simulink model "mj_res_test"  (R2025a)
settings: Solver=VariableStepAuto  StartTime=0.0  StopTime=2  RelTol=1e-3
undefined symbols (not defined in the file or in its folder): gray, zfar, znear
libraries: mjLib x3
settings Model: PacingRate=8  Creator=MuJoCo Simulink Blockset  LastModifiedBy=turbo
settings OptimizationCC: ReuseModelBlockBuffer=off
settings ModelReferenceCC: EnableRefExpFcnMdlSchedulingChecks=on
settings SFSimCC: SimTargetLang=C++  SimDLTargetLibrary=mkl-dnn
settings RTWCC: GPUComputeCapability=3.5

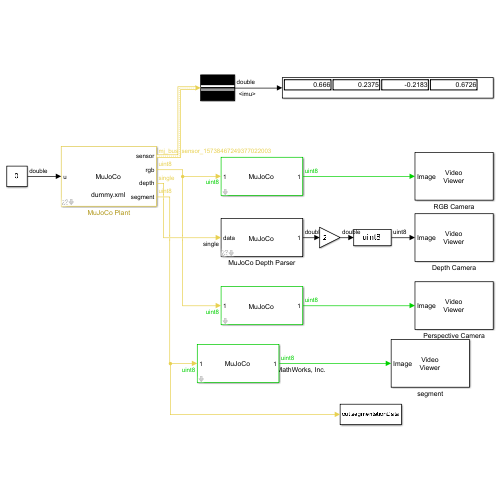
[thumbnail: Simulink's stored preview of the top-level diagram]
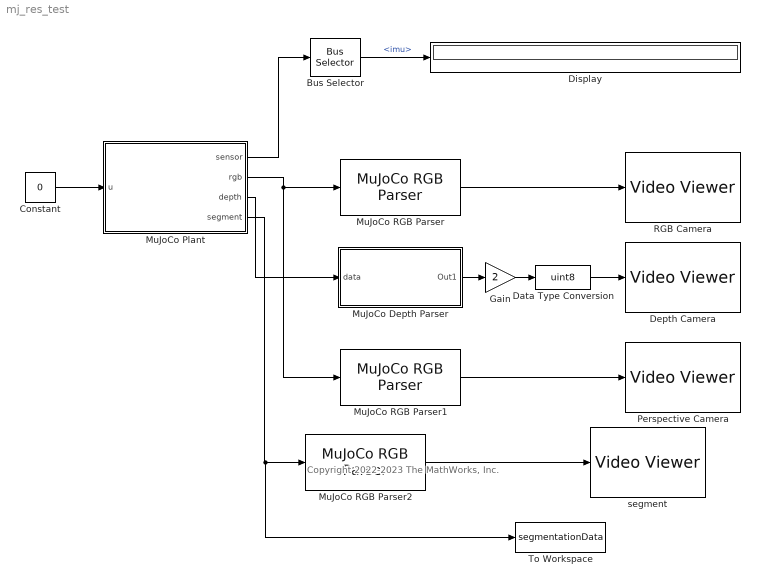
== system mj_res_test ==
  note: Copyright 2022-2023 The MathWorks, Inc.
  Bus Selector : BusSelector  OutputSignals=imu
  Constant : Constant  Value=0
  Data Type Conversion : DataTypeConversion  OutDataTypeStr=uint8  SaturateOnIntegerOverflow=off  RndMeth=Floor
  Depth Camera : VideoViewer  colormapValue=gray(256)  FigPos=[1776 885 418 465]
  Display : Display
  Gain : Gain  Gain=2
  MuJoCo Depth Parser : Subsystem  AncestorBlock=mjLib/MuJoCo Depth Parser  mask{inputBusType=mj_bus_rgb_3624495926710663437, selectedCamera=camera, imageRows=480, imageCols=640, startingIndex=307201, endingIndex=614400, orthographic_enable=on}
      mask prompts: inputBusType "Input Type"; selectedCamera "Select Camera"; orthographic_enable "Orthographic Camera"
      mask TypeOptions inputBusType: mj_bus_rgb_13812558253653659140
      mask Callback inputBusType:
      | inputBusType = get_param(gcb, 'inputBusType');
      | 
      | inputStruct = Simulink.Bus.createMATLABStruct(inputBusType);
      | 
      | mo = Simulink.Mask.get(gcb);
      | mo.Parameters(2).TypeOptions = fieldnames(inputStruct);
      mask TypeOptions selectedCamera: PerspectiveCamera | camera
      mask Callback selectedCamera:
      | inputBusType = get_param(gcb, 'inputBusType');
      | selectedCamera = get_param(gcb, 'selectedCamera');
      | 
      | inputStruct = Simulink.Bus.createMATLABStruct(inputBusType);
      | imageSize = size(inputStruct.(selectedCamera));
      | 
      | imageRows = imageSize(1);
      | imageCols = imageSize(2);
      | 
      | set_param(gcb, 'imageRows', num2str(imageRows));
      | set_param(gcb, 'imageCols', num2str(imageCols));
      | assignin('base', 'imageRows',imageRows);
      | assignin('base', 'imageCols',imageCols);
      | 
      | fields = fieldnames(inputStruct);
      | [~, camIndex] = ismember(selectedCamera, fields);
      | 
      | startingIndex = 1;
      | for i=1:(camIndex-1)
      |     imageSize = size(inputStruct.(fields{i}));
      |     startingIndex = startingIndex + imageSize(1)*imageSize(2);
      | end
      | endingIndex = startingIndex+imageSize(1) * imageSize(2) - 1;
      | 
      | set_param(gcb, 'startingIndex', num2str(startingIndex));
      | set_param(gcb, 'endingIndex', num2str(endingIndex));
      mask DialogControl Control2 Prompt: Refresh
      mask DialogControl Control2 Callback:
      | mo = Simulink.Mask.get(gcb);
      | mo.Parameters(1).TypeOptions = evalin('base', "who('mj_bus_rgb*')");
      mask Display:
      | color('black')
      | text(0.5, 0.5, 'MuJoCo', 'horizontalAlignment', 'center')
  MuJoCo Plant : Subsystem  AncestorBlock=mjLib/MuJoCo Plant  VariantControl=rgbOutOption  mask(MuJoCo Plant){controlBus=[], sensorBus=mj_bus_sensor_7979902499018342666, controlLength=[], sensorLength=[], rgbLength=[], depthLength=[], segLength=[], sampleTime=0.005, xmlFileRel=dummy.xml, xmlFile=dummy.xml, renderingType=Local, vsync=off, visualFPS=60, zoomLevel=1, keyframeName='home', znear=0.059256, zfar=296.2816, cameraSampleTime=0.020, rgbOutOption=on, depthOutOption=on, segmentationOutOption=on, customWidth=640, customHeight=480, specificCameraIndex=-1, controlInterfaceType=Vector}
      mask prompts: renderingType "Type"; visualFPS "FPS"; zoomLevel "Zoom"; keyframeName "Key Frame"; cameraSampleTime "Sample Time"; rgbOutOption "RGB Output"; depthOutOption "Depth Output"; segmentationOutOption "Segmentation Output"; customWidth "Width"; customHeight "Height"; specificCameraIndex "Camera Index"; controlInterfaceType "Interface"
      mask help:
      | This block provides an interface to MuJoCo™ physics engine.
      | It sets control inputs, steps the engine and outputs sensor/camera.
      |
      | Inputs, sensors, cameras and sample time information is obtained from the model XML.
      |
      | Control inputs are provided either as a non-virtual bus or vector.
      | Sensors are output as a non-virtual bus.
      | Camera data is output as a vector which can be decoded using MuJoCo RGB/Depth Parser blocks.
      mask init:
      | [controlBus, sensorBus, rgbBus, depthBus, segmentationBus, dataLengths] = mj_initbus(xmlFile);
      |     controlLength = double(dataLengths(1));
      |     sensorLength = double(dataLengths(2));
      |     rgbLength = double(dataLengths(3));
      |     depthLength = double(dataLengths(4));
      |     segLength = double(dataLengths(5));
      |     mj_maskinit;
      mask Callback xmlFileRel:
      | relpath = get_param(gcb, 'xmlFileRel');
      | 
      | abspath = which(relpath);
      | if isempty(abspath)
      |     abspath = relpath;
      | end
      | set_param(gcb, 'xmlFile', abspath);
      mask TypeOptions renderingType: Local | Global | None
      mask TypeOptions controlInterfaceType: Bus | Vector
      mask DialogControl Container3 Prompt: Model Info
      mask DialogControl controlBusText Prompt: Control Vector Type: [armMotor]
      mask DialogControl sensorBusText Prompt: Sensor Bus Type: mj_bus_sensor_15738467249377022003
      mask DialogControl rgbBusText Prompt: RGB Bus Type: mj_bus_rgb_3624495926710663437
      mask DialogControl depthBusText Prompt: Depth Bus Type: mj_bus_depth_3624495926710663437
      mask DialogControl segmentationBusText Prompt: Segmentation Bus Type: mj_bus_segmentation_3624495926710663437
      mask DialogControl sampleTimeText Prompt: Sample Time: 0.005
      mask DialogControl Container10 Prompt: Model
      mask DialogControl getFileButton Prompt: Browse
      mask DialogControl getFileButton Callback:
      | oldPath = get_param(gcb, 'xmlFile');
      | [file, path] = uigetfile({'*.xml;*.urdf'}, 'File Selector', oldPath);
      | if file~=0
      |     xml = fullfile(path, file);
      |     set_param(gcb, 'xmlFileRel', xml);
      | end
      mask DialogControl testStandaloneButton Prompt: Test
      mask DialogControl testStandaloneButton Callback:
      | % Get the absolute path of the XML file from the block parameter
      |     xmlFile = get_param(gcb, 'xmlFile');
      | 
      |     % Check if the XML file exists
      |     if ~isfile(xmlFile)
      |         error('The specified XML file does not exist: %s', xmlFile);
      |     end
      | 
      |     % Programmatically find the path to simulate.exe
      |     currentFilePath = mfilename('fullpath');
      |     [currentDir, ~, ~] = fileparts(currentFilePath);
      |     mujocoBinPath = fullfile(currentDir, '..', 'lib', 'win64', 'mujoco', 'bin');
      |     simulateExe = fullfile(mujocoBinPath, 'simulate.exe');
      | 
      |     % Check if simulate.exe exists
      |     if ~isfile(simulateExe)
      |         error('simulate.exe not found in the MuJoCo installation folder: %s', simulateExe);
      |     end
      | 
      |     % Run simulate.exe with the XML file as an argument
      |     command = sprintf('"%s" "%s"', simulateExe, xmlFile);
      |     disp(['Running command: ', command]);
      |     status = system(command);
      | 
      |     % Check the status of the command
      |     if status ~= 0
      |         error('Failed to run simulate.exe. Please check the XML file and MuJoCo installation.');
      |     else
      |         disp('Simulation completed successfully.');
      |     end
      mask DialogControl Container12 Prompt: Rendering
      mask DialogControl Control11 Prompt: Rendering thread is common to all MuJoCo blocks and is used for rendering visualizer window along with all cameras
      mask DialogControl Container9 Prompt: Visualizer
      mask DialogControl Control10 Prompt: Visualizer renders frames at specified FPS. Display buffer swap timing is controlled separately via vsync option.
      mask DialogControl renderingType Tooltip: Local rendering creates a unique window for each MuJoCo block. Global tries to merge different block visuals into one window. None disables visualization
      mask DialogControl Container11 Prompt: Options
      mask DialogControl vsync Tooltip: Vsync blocks rendering thread until the monitor is ready to show the next frame. This prevents screen tearing effect. Vsync can slow down everything including physics loop.
      mask DialogControl visualFPS Tooltip: If Vsync is disabled, specify the FPS to show visuals at.
      mask DialogControl Container13 Prompt: Camera
      mask DialogControl Control9 Prompt: Camera rendering runs in lockstep with physics engine.
      mask DialogControl rgbOutOption Tooltip: Render RGB camera
      mask DialogControl depthOutOption Tooltip: Disable depth buffer processing to improve simulation speed.
      mask DialogControl segmentationOutOption Tooltip: Enable segmentation image output using object IDs for each pixel.
      mask DialogControl Container7 Prompt: Control Inputs
      mask Display:
      | color('black')
      | text(0.5, 0.5, 'MuJoCo', 'horizontalAlignment', 'center')
      | [~, nameText, ext] = fileparts(get_param(gcb, 'xmlFile'));
      | text(0.5, 0.2, [nameText, ext], 'horizontalAlignment', 'center')
  MuJoCo RGB Parser : mjLib/MuJoCo RGB Parser  inputBusType=mj_bus_rgb_3624495926710663437  selectedCamera=camera  imageRows=480  imageCols=640  startingIndex=921601  endingIndex=1843200
      settings: SourceProductName=MuJoCo Simulator
  MuJoCo RGB Parser1 : mjLib/MuJoCo RGB Parser  inputBusType=mj_bus_rgb_3624495926710663437  selectedCamera=PerspectiveCamera  imageRows=480  imageCols=640  startingIndex=1  endingIndex=921600
      settings: SourceProductName=MuJoCo Simulator
  MuJoCo RGB Parser2 : mjLib/MuJoCo RGB Parser  inputBusType=mj_bus_rgb_3624495926710663437  selectedCamera=PerspectiveCamera  imageRows=480  imageCols=640  startingIndex=1  endingIndex=921600
      settings: SourceProductName=MuJoCo Simulator
  Perspective Camera : VideoViewer  colormapValue=gray(256)  FigPos=[551 807 418 304]
  RGB Camera : VideoViewer  FigPos=[1323 530 418 332]
  To Workspace : ToWorkspace  VariableName=segmentationData  SaveFormat=Timeseries  SampleTime=-1
  segment : VideoViewer  FigPos=[-428 1519 1118 553]
  wires:
  MuJoCo Plant/2(rgb) -> MuJoCo RGB Parser1/1, MuJoCo RGB Parser/1
  MuJoCo Plant/3(depth) -> MuJoCo Depth Parser/1(data)
  MuJoCo Plant/1(sensor) -> Bus Selector/1
  Bus Selector/1 -> Display/1  "<imu>"
  MuJoCo RGB Parser/1 -> RGB Camera/1
  MuJoCo Depth Parser/1(Out1) -> Gain/1
  Constant/1 -> MuJoCo Plant/1(u)
  Data Type Conversion/1 -> Depth Camera/1
  Gain/1 -> Data Type Conversion/1
  MuJoCo RGB Parser1/1 -> Perspective Camera/1
  MuJoCo RGB Parser2/1 -> segment/1
  MuJoCo Plant/4(segment) -> To Workspace/1, MuJoCo RGB Parser2/1

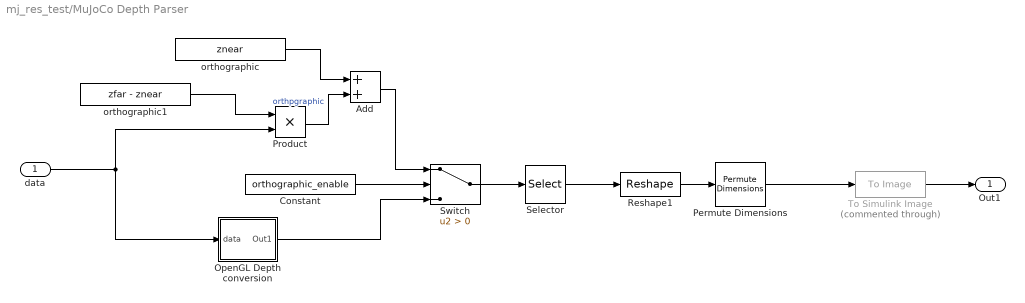
== system mj_res_test/MuJoCo Depth Parser ==
  data : Inport
  Add : Sum
  Constant : Constant  Value=orthographic_enable
  OpenGL Depth conversion : Subsystem
  Permute Dimensions : PermuteDimensions  Order=[3 2 1]
  Product : Product
  Reshape1 : Reshape  OutputDimensionality=Customize  OutputDimensions=[1,imageCols, imageRows]
  Selector : Selector  IndexOptions=Index vector (dialog)  Indices=startingIndex:endingIndex  OutputSizes=1
  Switch : Switch  Criteria=u2 > Threshold  SaturateOnIntegerOverflow=off  InputSameDT=off
  To Simulink Image : ToImage  Commented=through  OutDataTypeStr=Simulink.ImageType(imageRows,imageCols,1,'ColorFormat','Grayscale','Layout','ColumnMajor','ClassUnderlying','single')
  orthographic : Constant  Value=znear
  orthographic1 : Constant  Value=zfar - znear
  Out1 : Outport
  wires:
  Permute Dimensions/1 -> To Simulink Image/1
  To Simulink Image/1 -> Out1/1
  Selector/1 -> Reshape1/1
  data/1 -> OpenGL Depth conversion/1(data), Product/2
  Reshape1/1 -> Permute Dimensions/1
  Switch/1 -> Selector/1
  Constant/1 -> Switch/2
  orthographic1/1 -> Product/1
  OpenGL Depth conversion/1(Out1) -> Switch/3
  orthographic/1 -> Add/1
  Product/1 -> Add/2  "orthpgraphic"
  Add/1 -> Switch/1

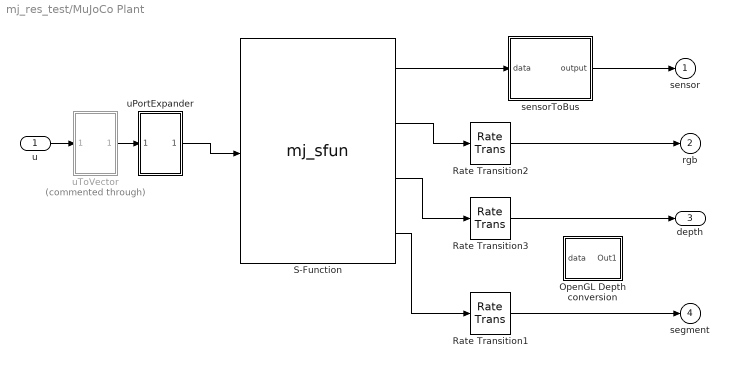
== system mj_res_test/MuJoCo Plant ==
  u : Inport  PortDimensions="[1  1]"
  OpenGL Depth conversion : Subsystem  AncestorBlock=mjLib/MuJoCo Depth Parser/OpenGL Depth conversion
  Rate Transition1 : RateTransition  OutPortSampleTime=cameraSampleTime
  Rate Transition2 : RateTransition  OutPortSampleTime=cameraSampleTime
  Rate Transition3 : RateTransition  OutPortSampleTime=cameraSampleTime
  S-Function : S-Function  FunctionName=mj_sfun  Parameters=xmlFile, renderingType, controlLength, sensorLength, rgbLength, depthLength, vsync, visualFPS, cameraSampleTime, sampleTime, zoomLevel,keyframeName, customWidth, customHeight, specificCameraIndex  SFunctionDeploymentMode=off  EnableBusSupport=off
  sensorToBus : Subsystem
  uPortExpander : Subsystem
  uToVector : Subsystem  Commented=through
  sensor : Outport
  rgb : Outport  Port=2
  depth : Outport  Port=3
  segment : Outport  Port=4
  wires:
  Rate Transition1/1 -> segment/1
  S-Function/4 -> Rate Transition1/1
  u/1 -> uToVector/1(In1)
  uToVector/1(Out1) -> uPortExpander/1(In1)
  S-Function/1 -> sensorToBus/1(data)
  sensorToBus/1(output) -> sensor/1
  uPortExpander/1(Out1) -> S-Function/1
  S-Function/2 -> Rate Transition2/1
  S-Function/3 -> Rate Transition3/1
  Rate Transition2/1 -> rgb/1
  Rate Transition3/1 -> depth/1

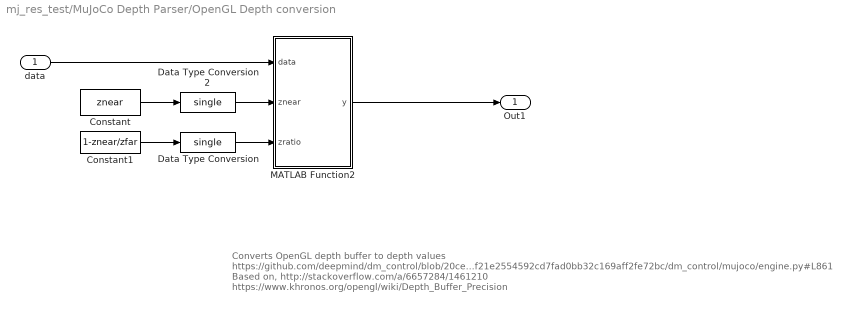
== system mj_res_test/MuJoCo Depth Parser/OpenGL Depth conversion ==
  note: Converts OpenGL depth buffer to depth values
      | https://github.com/deepmind/dm_control/blob/20cef21e2554592cd7fad0bb32c169aff2fe72bc/dm_control/mujoco/engine.py#L861
      | Based on,
      | http://stackoverflow.com/a/6657284/1461210
      | https://www.khronos.org/opengl/wiki/Depth_Buffer_Precision
  data : Inport
  Constant : Constant  Value=znear
  Constant1 : Constant  Value=1-znear/zfar
  Data Type Conversion : DataTypeConversion  OutDataTypeStr=single  SaturateOnIntegerOverflow=off  RndMeth=Floor
  Data Type Conversion2 : DataTypeConversion  OutDataTypeStr=single  SaturateOnIntegerOverflow=off  RndMeth=Floor
  MATLAB Function2 : MATLAB Function  TreatAsAtomicUnit=on
  Out1 : Outport
  wires:
  Constant/1 -> Data Type Conversion2/1
  Constant1/1 -> Data Type Conversion/1
  Data Type Conversion2/1 -> MATLAB Function2/2(znear)
  data/1 -> MATLAB Function2/1(data)
  Data Type Conversion/1 -> MATLAB Function2/3(zratio)
  MATLAB Function2/1(y) -> Out1/1

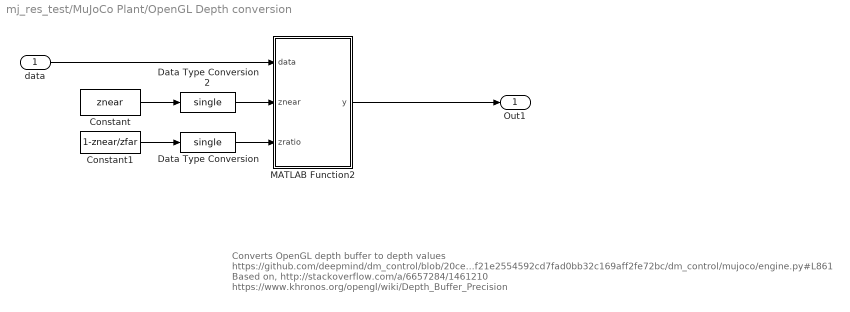
== system mj_res_test/MuJoCo Plant/OpenGL Depth conversion ==
  note: Converts OpenGL depth buffer to depth values
      | https://github.com/deepmind/dm_control/blob/20cef21e2554592cd7fad0bb32c169aff2fe72bc/dm_control/mujoco/engine.py#L861
      | Based on,
      | http://stackoverflow.com/a/6657284/1461210
      | https://www.khronos.org/opengl/wiki/Depth_Buffer_Precision
  data : Inport
  Constant : Constant  Value=znear
  Constant1 : Constant  Value=1-znear/zfar
  Data Type Conversion : DataTypeConversion  OutDataTypeStr=single  SaturateOnIntegerOverflow=off  RndMeth=Floor
  Data Type Conversion2 : DataTypeConversion  OutDataTypeStr=single  SaturateOnIntegerOverflow=off  RndMeth=Floor
  MATLAB Function2 : MATLAB Function  TreatAsAtomicUnit=on
  Out1 : Outport
  wires:
  Constant/1 -> Data Type Conversion2/1
  Constant1/1 -> Data Type Conversion/1
  Data Type Conversion2/1 -> MATLAB Function2/2(znear)
  data/1 -> MATLAB Function2/1(data)
  Data Type Conversion/1 -> MATLAB Function2/3(zratio)
  MATLAB Function2/1(y) -> Out1/1

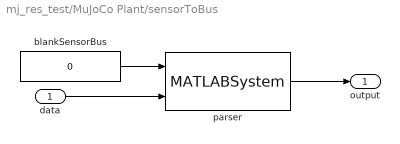
== system mj_res_test/MuJoCo Plant/sensorToBus ==
  data : Inport
  blankSensorBus : Constant  Value=0  OutDataTypeStr=Bus: mj_bus_sensor_15738467249377022003
  parser : MATLABSystem  System=mj_sensor_parser  OutputBusName=mj_bus_sensor_15738467249377022003  SimulateUsing=Code generation
      mask Type: mj_sensor_parser
  output : Outport
  wires:
  blankSensorBus/1 -> parser/1
  data/1 -> parser/2
  parser/1 -> output/1

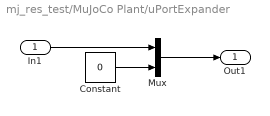
== system mj_res_test/MuJoCo Plant/uPortExpander ==
  In1 : Inport
  Constant : Constant  Value=0
  Mux : Mux  Inputs=2
  Out1 : Outport
  wires:
  In1/1 -> Mux/1
  Mux/1 -> Out1/1
  Constant/1 -> Mux/2

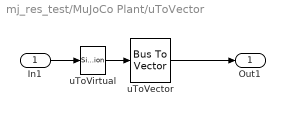
== system mj_res_test/MuJoCo Plant/uToVector ==
  In1 : Inport
  uToVector : BusToVector
  uToVirtual : SignalConversion  ConversionOutput=Virtual bus  OverrideOpt=off
  Out1 : Outport
  wires:
  uToVirtual/1 -> uToVector/1
  In1/1 -> uToVirtual/1
  uToVector/1 -> Out1/1

== matlab function mj_res_test/MuJoCo Depth Parser/OpenGL Depth conversion/MATLAB Function2 ==
  data: data input; znear input; zratio input; y output
function y = fcn(data, znear, zratio)
y = znear./(1-data*zratio);

== matlab function mj_res_test/MuJoCo Plant/OpenGL Depth conversion/MATLAB Function2 ==
  data: data input; znear input; zratio input; y output
function y = fcn(data, znear, zratio)
y = znear./(1-data*zratio);
